simulink model "PIDcon"  (Simulink 7.6)
settings: Solver=ode23  StartTime=0.0  StopTime=100.0  RelTol=1e-3
settings Model: Creator=Administrator  LastModifiedBy=Administrator
settings OptimizationCC: InitFltsAndDblsToZero=on
settings DebuggingCC: SaveWithParameterizedLinksMsg=none  SignalResolutionControl=TryResolveAllWithWarning  MultiTaskDSMMsg=warning  MultiTaskCondExecSysMsg=none  StrictBusMsg=None
settings RTWCC: IncludeERTFirstTime=on
settings GRTTargetCC: TargetFcnLib=ansi_tfl_tmw.mat

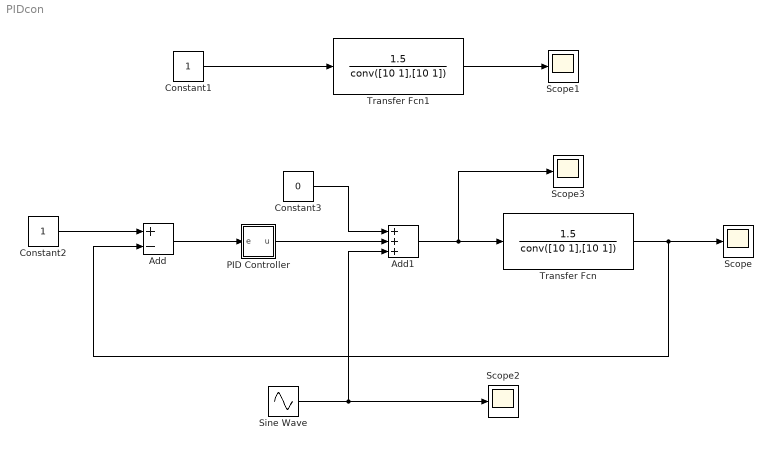
== system PIDcon ==
  Add : Sum  Inputs=+-
  Add1 : Sum  Inputs=+++
  Constant1 : Constant
  Constant2 : Constant
  Constant3 : Constant  Value=0
  PID Controller : Subsystem  AncestorBlock=simulink_need_slupdate/PID Controller  mask(PID Controller){P=8, I=0.01, D=0}
      mask prompts: P "Proportional:"; I "Integral:"; D "Derivative:"
      mask help:
      | Enter expressions for proportional, integral, and derivative terms.
      | P+I/s+Ds
      mask Help: This block implements a PID controller where parameters are entered for the Proportional, Integral and Derivative terms. Unmask this block to see how it works. The derivative term is implemented using a true derivative block.
      mask Display: disp('PID')
  Scope{,1..3} (4 alike) : Scope
      Scope1 settings: TimeRange=100
      Scope2 settings: SaveName=ScopeData2
      Scope3 settings: TimeRange=100  SaveName=ScopeData3
  Sine Wave : Sin  Amplitude=0  SampleTime=0
  Transfer Fcn : TransferFcn  Numerator=[1.5]  Denominator=conv([10 1],[10 1])
  Transfer Fcn1 : TransferFcn  Numerator=[1.5]  Denominator=conv([10 1],[10 1])
  wires:
  Add/1 -> PID Controller/1(e)
  Transfer Fcn/1 -> Scope/1, Add/2
  Constant1/1 -> Transfer Fcn1/1
  Transfer Fcn1/1 -> Scope1/1
  Add1/1 -> Transfer Fcn/1, Scope3/1
  PID Controller/1(u) -> Add1/2
  Constant3/1 -> Add1/1
  Sine Wave/1 -> Add1/3, Scope2/1
  Constant2/1 -> Add/1

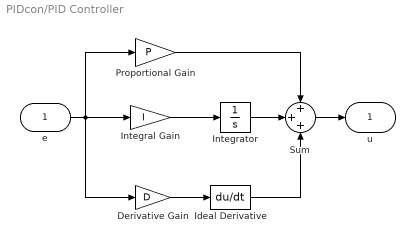
== system PIDcon/PID Controller ==
  e : Inport
  Derivative Gain : Gain  Gain=D  SaturateOnIntegerOverflow=on  OutDataTypeStr=Inherit: Same as input  ParamDataTypeStr=Inherit: Same as input
  Ideal Derivative : Derivative
  Integral Gain : Gain  Gain=I  SaturateOnIntegerOverflow=on  OutDataTypeStr=Inherit: Same as input  ParamDataTypeStr=Inherit: Same as input
  Integrator : Integrator
  Proportional Gain : Gain  Gain=P  SaturateOnIntegerOverflow=on  OutDataTypeStr=Inherit: Same as input  ParamDataTypeStr=Inherit: Same as input
  Sum : Sum  Inputs=+++  SaturateOnIntegerOverflow=on  InputSameDT=on  OutDataTypeStr=Inherit: Same as first input
  u : Outport  InitialOutput=0
  wires:
  Integral Gain/1 -> Integrator/1
  Proportional Gain/1 -> Sum/1
  Integrator/1 -> Sum/2
  Ideal Derivative/1 -> Sum/3
  e/1 -> Derivative Gain/1, Proportional Gain/1, Integral Gain/1
  Sum/1 -> u/1
  Derivative Gain/1 -> Ideal Derivative/1
